simulink model "Sim8_03_test_Gfe_PI"  (R2020b)
settings: Solver=ode1  StartTime=0.0  StopTime=10  FixedStep=Time_Step  MaxStep=1e-4  RelTol=1e-3
undefined symbols (not defined in the file): Bxx_GenericVoltageSource, H_dc, Lg, P_dcb, Rg, Source_Lib, Theta0, Time_Step, Udc_n, Un, V0
libraries: spsBreakerLib x6, Control_Lib x6, spsThreePhaseSourceLib x4, spsControlledVoltageSourceLib x3, spsGroundLib x2, spsLoadFlowBusLib x2, spsThreePhaseVIMeasurementLib x2, spsThreePhaseBreakerLib x2, spsVoltageMeasurementLib x2, spsSeriesRLCBranchLib x2, spsControlledCurrentSourceLib x1, spsUniversalBridgeLib x1
(part 2 of 2)

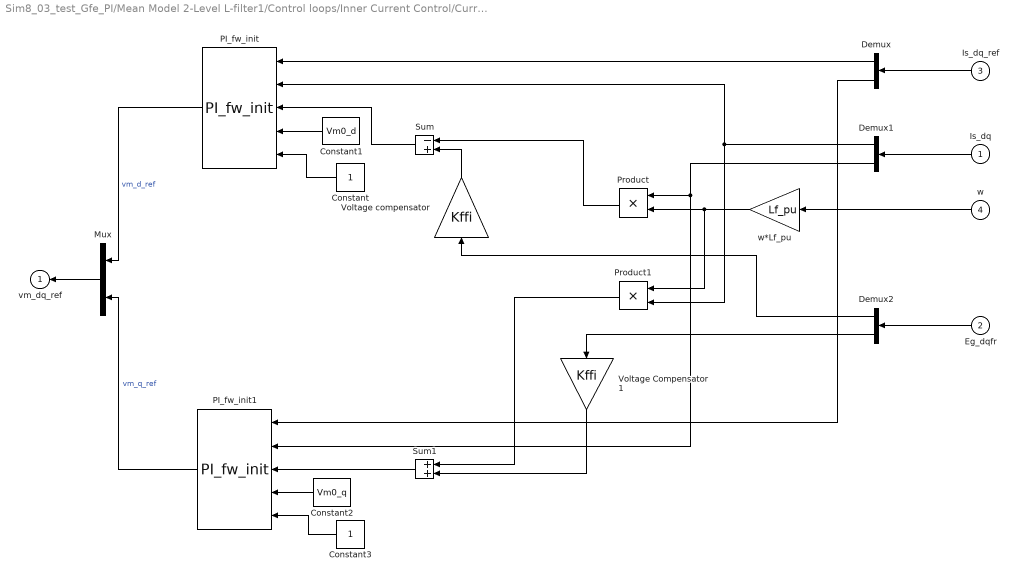
== system Sim8_03_test_Gfe_PI/Mean Model 2-Level L-filter1/Control loops/Inner Current Control/Current PI control ==
  Is_dq : Inport
  Eg_dqfr : Inport  Port=2
  Is_dq_ref : Inport  Port=3
  w : Inport  Port=4
  Constant : Constant
  Constant1 : Constant  Value=Vm0_d
  Constant2 : Constant  Value=Vm0_q
  Constant3 : Constant
  Demux : Demux  Outputs=2
  Demux1 : Demux  Outputs=2
  Demux2 : Demux  Outputs=2
  Mux : Mux  Inputs=[1 1]
  PI_fw_init : Control_Lib/PI_fw_init  Kp=Kp_i  Ki=Ki_i
      settings: SourceProductName=VSC4SPS
  PI_fw_init1 : Control_Lib/PI_fw_init  Kp=Kp_i  Ki=Ki_i
      settings: SourceProductName=VSC4SPS
  Product : Product  RndMeth=Zero
  Product1 : Product  RndMeth=Zero
  Sum : Sum  Inputs=-+
  Sum1 : Sum
  Voltage Compensator 1 : Gain  Gain=Kffi
  Voltage compensator : Gain  Gain=Kffi
  w*Lf_pu : Gain  Gain=Lf_pu
  vm_dq_ref : Outport  InitialOutput=0  VectorParamsAs1DForOutWhenUnconnected=off
  wires:
  Constant3/1 -> PI_fw_init1/5
  Constant2/1 -> PI_fw_init1/4
  Voltage Compensator 1/1 -> Sum1/2
  Sum1/1 -> PI_fw_init1/3
  Constant1/1 -> PI_fw_init/4
  Constant/1 -> PI_fw_init/5
  Sum/1 -> PI_fw_init/3
  Product/1 -> Sum/1
  Eg_dqfr/1 -> Demux2/1
  Demux2/2 -> Voltage Compensator 1/1
  Demux2/1 -> Voltage compensator/1
  Is_dq/1 -> Demux1/1
  Is_dq_ref/1 -> Demux/1
  Demux/1 -> PI_fw_init/1
  Demux1/1 -> Product1/2, PI_fw_init/2
  w*Lf_pu/1 -> Product1/1, Product/2
  Demux1/2 -> Product/1, PI_fw_init1/2
  Mux/1 -> vm_dq_ref/1
  Demux/2 -> PI_fw_init1/1
  Product1/1 -> Sum1/1
  PI_fw_init/1 -> Mux/1  "vm_d_ref"
  PI_fw_init1/1 -> Mux/2  "vm_q_ref"
  w/1 -> w*Lf_pu/1
  Voltage compensator/1 -> Sum/2
